simulink model "hdv_hydroelectropowertrain_model"  (R2026a)
settings: Solver=ode1be  StopTime=simulation_length  FixedStep=tsample  MaxStep=tsample
undefined symbols (not defined in the file): alpha, Apump, available_torque, Bpump, btheta_shaft, C1, consumption, Cpump, dp_lim, E0, E1, E2, E3, E_1, Elog, eta_v_m, eta_v_p, ki_dp_comp, ki_te_comp, kp_ctrl_m, kp_dp_comp, kp_te_comp, Kpump, load_blade_enable, Lpump, M, magnitude, Ncell, Npump, omega_e_rpm_ref, omega_l_max_rpm, q1Kalman, q2Kalman, q3Kalman, Qhr, R0, R1, R_tg, rKalman, rpm_base, rpm_consumption, simulation_length, tau_load, tau_load_max, Tc, torque_base, torque_consumption, torque_friction_base, tsample, v_track1_ref, v_track2_ref, valve_mmorifice_max, xv_m_max
libraries: fl_lib x383, nesl_utility x162, linear_swashplate_ctrl_lib x8, flexshaft_lib x5, bichamber_piston_lib x5, variable_displacement_motor_lib x4, variable_displacement_pump_lib x4, fixed_displacement_pump_lib x4, relief_valve_lib x4, inverse_shuttle_valve_lib x4, hydrostatic_threeway_valve_bichamber_piston_lib x4, hydrostatic_fourway_valve_bichamber_piston_lib x4
(part 3 of 8)

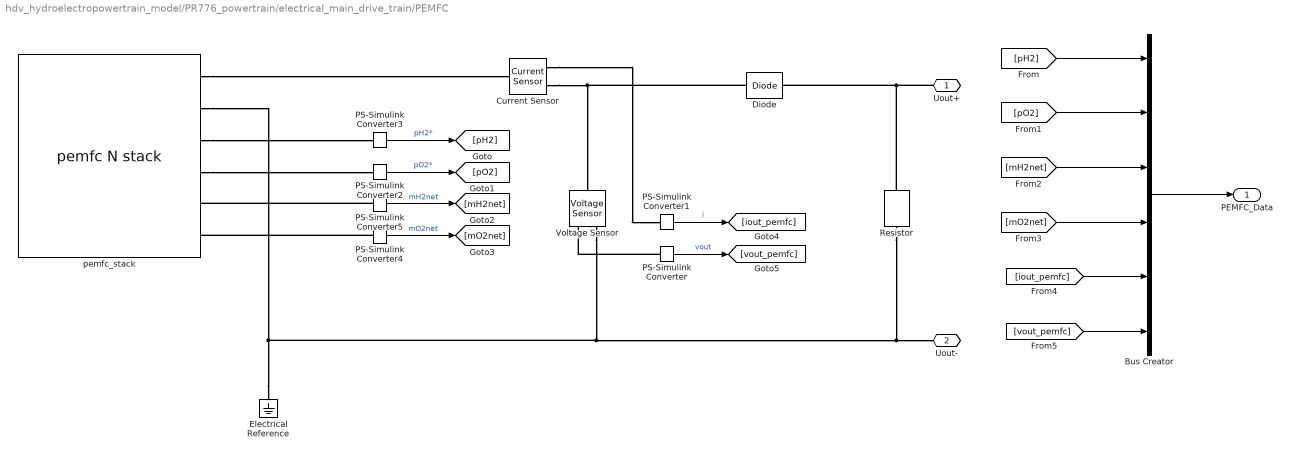
== system hdv_hydroelectropowertrain_model/PR776_powertrain/electrical_main_drive_train/PEMFC ==
  Bus Creator : BusCreator  Inputs=6
  Current Sensor : fl_lib/Electrical/Electrical Sensors/Current Sensor
  Diode : ee_lib/Semiconductors & Converters/Diode  ModelType=ee.enum.diode.modelType.pwl  TableType=ee.enum.diode.tableType.IfMat  IfMat=[.07, .12, .19, 1.75, 4.24, 7.32, 11.2; .16, .3, .72, 2.14, 5.02, 8.35, 13.12] A  VfMat=[.9, 1.15, 1.25, 1.5, 1.75, 2.17, 2.6, 2.85; .58, .68, .75, 1.1, 1.38, 1.77, 2.27, 2.7] V  TjVec=[25, 125] degC  VfVec=[.5, .7, .9, 1.3, 1.7, 2.1, 2.5] V  IfVec=[.1, .2, .5, 1, 2, 4, 7, 10] A  IrMat=[1e-06, 2e-06, 5e-06, 1e-05, 2.5e-05, 5e-05, .0001; 2e-06, 5e-06, 1e-05, 4e-05, 8e-05, .0002, .0005] A  VrMat=[10, 100, 200, 250, 300, 325, 350; 10, 70, 160, 220, 270, 300, 320] V  VrVec=[10, 20, 40, 50, 70, 80, 100] V  IrVec=[1e-06, 2e-06, 5e-06, 1e-05, 2e-05, 5e-05, .0001] A  Vf=0.6 V  Ron=0.3 Ohm  Goff=1e-8 S  prmExp=ee.enum.diode.expParam.useTwo  I12=[.0137, .545] A  V12=[.6, .7] V  RS=0 Ohm  Tmeas=25 degC  IS=1e-12 A  ec=1  I1=0.0137 A  V1=0.6 V  N_series=1  N_parallel=1  ZenerEnable=false  Rz=0.3 Ohm  BV=inf V  C_param=ee.enum.diode.capParam.fixed  CJ=5 pF  CJ0=5 pF  Vvec=[.1, 10, 100] V  Cvec=[3.5, 1, .4] pF  VJ=1 V  Mgrad=0.5  FC=0.5  Q_param=ee.enum.diode.recoveryParam.off  iRM=-7.15 A  iF=4 A  didt=-750 A/us  trr_factor=3  trr=115 ns  Qrr=1500 s*uA  Vr=-600 V  Ls=150 nH  Erec=0.03 J  TT=50 ns  tau=100 ns  T_param=ee.enum.diode.temperatureParam.off  Tdevice=25 degC  I1_T2=0.245 A  V1_T2=0.5 V  IS_T2=1.25e-7 A  Tmeas2=125 degC  XTI_param=ee.enum.diode.xtiParam.pn  XTI=3  EG_param=ee.enum.diode.egapParam.material_si  EG=1.11 eV  dBVdT=0 V/K  enable_fault_input=simscape.enum.onoff.off  i_specify=off  i_priority=None  i=0 A  i_nominal_specify=off  i_nominal_value=1  i_nominal_unit=A  v_specify=off  v_priority=None  v=0 V  v_nominal_specify=off  v_nominal_value=1  v_nominal_unit=V  v_capacitor_specify=off  v_capacitor_priority=None  v_capacitor=0 V  v_capacitor_nominal_specify=off  v_capacitor_nominal_value=1  v_capacitor_nominal_unit=V  Qj_specify=off  Qj_priority=High  Qj=0 C  Qj_nominal_specify=off  Qj_nominal_value=1  Qj_nominal_unit=C  i_diode_specify=off  i_diode_priority=None  i_diode=0 A  i_diode_nominal_specify=off  i_diode_nominal_value=1  i_diode_nominal_unit=A  v_diode_specify=off  v_diode_priority=None  v_diode=0 V  v_diode_nominal_specify=off  v_diode_nominal_value=1  v_diode_nominal_unit=V  i_capacitor_specify=off  i_capacitor_priority=None  i_capacitor=0 A  i_capacitor_nominal_specify=off  i_capacitor_nominal_value=1  i_capacitor_nominal_unit=A  fidelity_level=ee.enum.diode.fidelity.includeChargeDyn  rec_loss_model=ee.enum.diode.reverseRecoveryModel.fixed  ErecVal=0 J  scaleWithIandV=true  ErecMat=zeros(2, 3) J  ErecMat3D=zeros(2, 3, 2) J  TjrecVec=[298.15, 398.15] K  IfrecVec=[.1, 1, 10] A  IrecVal=10 A  VrecVal=10 V  VrecVec=[0, 100] V  tFilter=1 / 1000 / 100 s  thermal_network_parameterization=ee.enum.thermalNetworkTopology.junctionCase  Rth=[0, 10] K/W  Rth_Cauer=[1, 3, 10] K/W  Rth_Foster=[4, 6] K/W  thermal_mass_parameterization=ee.enum.thermalNetwork.timeconstant  thermal_mass=[0, 1] J/K  thermal_mass_Cauer=[.1, .3, 1] J/K  thermal_mass_Foster=[1.5, 3] J/K  thermal_time_constant=[0, 10] s  thermal_time_constant_Cauer=[1, 3, 10] s  thermal_time_constant_Foster=[6, 18] s  thermal_mass_initial_temperatures=[25, 25] degC  thermal_mass_initial_temperatures_Cauer=[25, 25, 25] degC  junction_thermal_mass=0.01 J/K  Tvec_initial_Foster=[25, 25, 25, 25] degC  no_thermal_network=0  junction_temperature_specify=off  junction_temperature_priority=None  junction_temperature=25 degC  junction_temperature_nominal_specify=off  junction_temperature_nominal_value=1  junction_temperature_nominal_unit=degC
  Electrical Reference : fl_lib/Electrical/Electrical Elements/Electrical Reference
  PS-Simulink Converter{,1..5} (6 alike) : nesl_utility/PS-Simulink Converter  PhysicalDomain=network_engine_domain  SubClassName=ps_output  LeftPortType=input  RightPortType=output  PseudoPeriodic=off  Frequencies=[]  VectorFormat=1-D array  Unit=inherit  AffineConversion=off
  Resistor : fl_lib/Electrical/Electrical Elements/Resistor  R=1e2 Ohm  i_specify=off  i_priority=None  i=0 A  i_nominal_specify=off  i_nominal_value=1  i_nominal_unit=A  v_specify=off  v_priority=None  v=0 V  v_nominal_specify=off  v_nominal_value=1  v_nominal_unit=V
  Voltage Sensor : fl_lib/Electrical/Electrical Sensors/Voltage Sensor
  pemfc_stack : pemfc_stack_lib/pemfc N stack  F=96487 s*A/mol  R=8.314 J/K/mol  T=298 K  DGibbs=285800 J/mol  n=2  Va=Va m^3  Vc=Vc m^3  tau_a=0.15 s  tau_c=0.15 s  p0=1e5 Pa  Ncells=Ncells  Rohm0=Rohm0 Ohm  Ract=Ract Ohm  Rconc=Rconc Ohm  Cdlc=Cdlc F  e_specify=off  e_priority=None  e=0 V  e_nominal_specify=off  e_nominal_unit=V  e_nominal_value=1  u_specify=off  u_priority=None  u=0 V  u_nominal_specify=off  u_nominal_unit=V  u_nominal_value=1  uc_specify=off  uc_priority=None  uc=0 V  uc_nominal_specify=off  uc_nominal_unit=V  uc_nominal_value=1  icell_specify=off  icell_priority=None  icell=0 A  icell_nominal_specify=off  icell_nominal_unit=A  icell_nominal_value=1  pH2_star_specify=off  pH2_star_priority=High  pH2_star=3  pH2_star_nominal_specify=off  pH2_star_nominal_unit=1  pH2_star_nominal_value=1  pO2_star_specify=off  pO2_star_priority=High  pO2_star=3  pO2_star_nominal_specify=off  pO2_star_nominal_unit=1  pO2_star_nominal_value=1  mH2_net_specify=off  mH2_net_priority=None  mH2_net=0 mol/s  mH2_net_nominal_specify=off  mH2_net_nominal_unit=mol/s  mH2_net_nominal_value=1  mO2_net_specify=off  mO2_net_priority=None  mO2_net=0 mol/s  mO2_net_nominal_specify=off  mO2_net_nominal_unit=mol/s  mO2_net_nominal_value=1  mask(pemfc N stack){}
  Uout+ : PMIOPort  Side=Right
  Uout- : PMIOPort  Port=2  Side=Right
  PEMFC_Data : Outport
  wires:
  PS-Simulink Converter2/1 -> [pO2]  "pO2*"
  PS-Simulink Converter1/1 -> [iout_pemfc]  "i"
  PS-Simulink Converter/1 -> [vout_pemfc]  "vout"
  PS-Simulink Converter3/1 -> [pH2]  "pH2*"
  PS-Simulink Converter5/1 -> [mH2net]  "mH2net"
  PS-Simulink Converter4/1 -> [mO2net]  "mO2net"
  Bus Creator/1 -> PEMFC_Data/1
  [pH2] -> Bus Creator/1
  [vout_pemfc] -> Bus Creator/6
  [pO2] -> Bus Creator/2
  [mH2net] -> Bus Creator/3
  [mO2net] -> Bus Creator/4
  [iout_pemfc] -> Bus Creator/5
  connections:
  pemfc_stack/RConn3 -- PS-Simulink Converter3/LConn1
  PS-Simulink Converter/LConn1 -- Voltage Sensor/RConn1
  pemfc_stack/RConn1 -- Current Sensor/LConn1
  pemfc_stack/RConn4 -- PS-Simulink Converter2/LConn1
  Electrical Reference/LConn1 -- Voltage Sensor/RConn2 -- Resistor/RConn1 -- Uout-/RConn1 -- pemfc_stack/RConn2
  Current Sensor/RConn1 -- PS-Simulink Converter1/LConn1
  PS-Simulink Converter4/LConn1 -- pemfc_stack/RConn6
  PS-Simulink Converter5/LConn1 -- pemfc_stack/RConn5
  Current Sensor/RConn2 -- Diode/LConn1 -- Voltage Sensor/LConn1
  Resistor/LConn1 -- Uout+/RConn1 -- Diode/RConn1

== system hdv_hydroelectropowertrain_model/PR776_powertrain/electrical_main_drive_train/battery_management ==
  vout(k) : Inport
  i(k) : Inport  Port=2
  Constant : Constant  Value=tsample
  Constant1 : Constant  Value=Qhr
  Constant2 : Constant  Value=q1Kalman
  Constant3 : Constant  Value=q2Kalman
  Constant4 : Constant  Value=q3Kalman
  Constant5 : Constant  Value=rKalman
  Constant6 : Constant  Value=tsample
  Constant7 : Constant  Value=Qhr
  Selector : Selector  InputPortWidth=3  IndexOptions=Index vector (dialog)  Indices=1  OutputSizes=1
  Unit Delay4 : UnitDelay  SampleTime=tsample
  kalman_observer_gains : MATLAB Function  TreatAsAtomicUnit=on  SystemSampleTime=tsample
  lithium-ion battery model : MATLAB Function  TreatAsAtomicUnit=on  SystemSampleTime=tsample
  SOC(k) : Outport
  vout_hat : Outport  Port=2
  wires:
  lithium-ion battery model/1(SOC) -> SOC(k)/1  "SOC"
  Constant6/1 -> kalman_observer_gains/2(ts)
  vout(k)/1 -> lithium-ion battery model/7(vout)
  kalman_observer_gains/2(l2) -> lithium-ion battery model/5(l2)
  Selector/1 -> Unit Delay4/1
  kalman_observer_gains/3(l3) -> lithium-ion battery model/6(l3)
  kalman_observer_gains/1(l1) -> lithium-ion battery model/4(l1)
  Constant7/1 -> kalman_observer_gains/8(Qhr)
  Constant1/1 -> lithium-ion battery model/3(Qhr)
  Constant5/1 -> kalman_observer_gains/7(r)
  Constant4/1 -> kalman_observer_gains/6(q3)
  Constant2/1 -> kalman_observer_gains/4(q1)
  Constant/1 -> lithium-ion battery model/2(ts)
  i(k)/1 -> kalman_observer_gains/1(iz), lithium-ion battery model/1(iz)
  lithium-ion battery model/3(x) -> Selector/1  "x(k+1|k)"
  Unit Delay4/1 -> kalman_observer_gains/3(z)  "x(k|k-1)"
  Constant3/1 -> kalman_observer_gains/5(q2)
  lithium-ion battery model/2(u) -> vout_hat/1  "vout_hat"

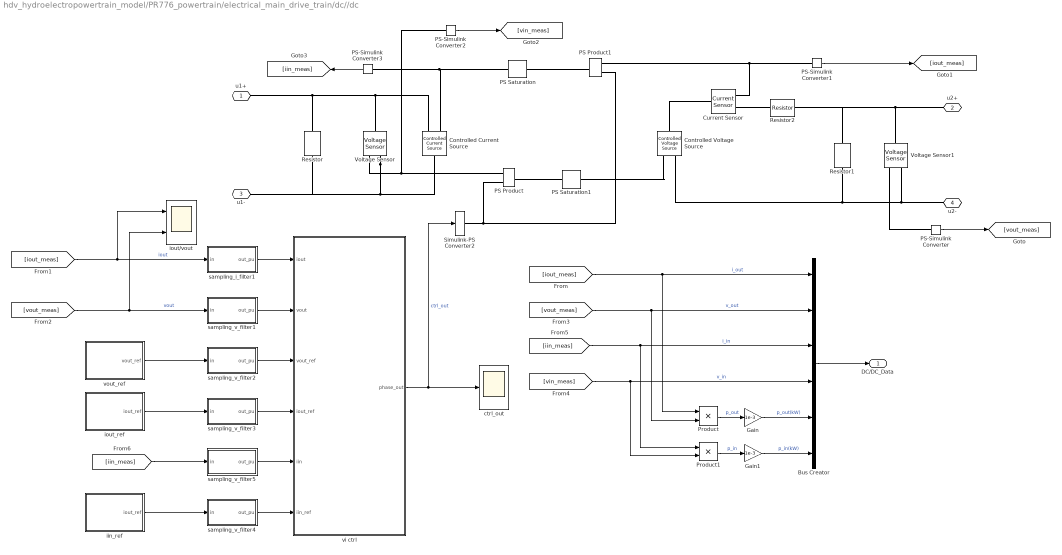
== system hdv_hydroelectropowertrain_model/PR776_powertrain/electrical_main_drive_train/dc//dc ==
  Bus Creator : BusCreator  Inputs=6
  Controlled Current Source : fl_lib/Electrical/Electrical Sources/Controlled Current Source
  Controlled Voltage Source : fl_lib/Electrical/Electrical Sources/Controlled Voltage Source
  Current Sensor : fl_lib/Electrical/Electrical Sensors/Current Sensor
  Gain : Gain  Gain=1e-3
  Gain1 : Gain  Gain=1e-3
  PS Product : fl_lib/Physical Signals/Functions/PS Product
  PS Product1 : fl_lib/Physical Signals/Functions/PS Product
  PS Saturation : fl_lib/Physical Signals/Nonlinear Operators/PS Saturation  upper_limit=inf A  lower_limit=-inf A  ZeroCross=true
  PS Saturation1 : fl_lib/Physical Signals/Nonlinear Operators/PS Saturation  upper_limit=inf V  lower_limit=-inf V  ZeroCross=true
  PS-Simulink Converter : nesl_utility/PS-Simulink Converter  PhysicalDomain=network_engine_domain  SubClassName=ps_output  LeftPortType=input  RightPortType=output  PseudoPeriodic=off  Frequencies=[]  VectorFormat=1-D array  Unit=inherit  AffineConversion=off
  PS-Simulink Converter1 : nesl_utility/PS-Simulink Converter  PhysicalDomain=network_engine_domain  SubClassName=ps_output  LeftPortType=input  RightPortType=output  PseudoPeriodic=off  Frequencies=[]  VectorFormat=1-D array  Unit=inherit  AffineConversion=on
  PS-Simulink Converter2 : nesl_utility/PS-Simulink Converter  PhysicalDomain=network_engine_domain  SubClassName=ps_output  LeftPortType=input  RightPortType=output  PseudoPeriodic=off  Frequencies=[]  VectorFormat=1-D array  Unit=inherit  AffineConversion=off
  PS-Simulink Converter3 : nesl_utility/PS-Simulink Converter  PhysicalDomain=network_engine_domain  SubClassName=ps_output  LeftPortType=input  RightPortType=output  PseudoPeriodic=off  Frequencies=[]  VectorFormat=1-D array  Unit=inherit  AffineConversion=off
  Product : Product
  Product1 : Product
  Resistor : fl_lib/Electrical/Electrical Elements/Resistor  R=1e4 Ohm  i_specify=off  i_priority=None  i=0 A  i_nominal_specify=off  i_nominal_value=1  i_nominal_unit=A  v_specify=off  v_priority=None  v=0 V  v_nominal_specify=off  v_nominal_value=1  v_nominal_unit=V
  Resistor1 : fl_lib/Electrical/Electrical Elements/Resistor  R=1e4 Ohm  i_specify=off  i_priority=None  i=0 A  i_nominal_specify=off  i_nominal_value=1  i_nominal_unit=A  v_specify=off  v_priority=None  v=0 V  v_nominal_specify=off  v_nominal_value=1  v_nominal_unit=V
  Resistor2 : fl_lib/Electrical/Electrical Elements/Resistor  R=5e-3 Ohm  i_specify=off  i_priority=None  i=0 A  i_nominal_specify=off  i_nominal_value=1  i_nominal_unit=A  v_specify=off  v_priority=None  v=0 V  v_nominal_specify=off  v_nominal_value=1  v_nominal_unit=V
  Simulink-PS Converter2 : nesl_utility/Simulink-PS Converter  PhysicalDomain=network_engine_domain  SubClassName=ps_input  LeftPortType=input  RightPortType=output  PseudoPeriodic=off  Frequencies=[]  NoiseDistribution=none  NoiseParameters=[]  Unit=1  AffineConversion=on  FilteringAndDerivatives=zero  SimscapeFilterOrder=2  InputFilterTimeConstant=tsample  UdotUserProvided=2
  Voltage Sensor : fl_lib/Electrical/Electrical Sensors/Voltage Sensor
  Voltage Sensor1 : fl_lib/Electrical/Electrical Sensors/Voltage Sensor
  ctrl_out : Scope
      settings: ActiveDisplayYMinimum=-0.85725  ActiveDisplayYMaximum=7.71521  DataLoggingVariableName=ScopeData5
  iin_ref : Subsystem
  iout/vout : Scope  NumInputPorts=2
      settings: ActiveDisplayYMinimum=-127511.09356  ActiveDisplayYMaximum=14266.88646
  iout_ref : Subsystem
  sampling_i_filter1 : Subsystem
  sampling_v_filter1 : Subsystem
  sampling_v_filter2 : Subsystem
  sampling_v_filter3 : Subsystem
  sampling_v_filter4 : Subsystem
  sampling_v_filter5 : Subsystem
  vi ctrl : Subsystem
  vout_ref : Subsystem
  u1+ : PMIOPort  Side=Left
  u2+ : PMIOPort  Port=2  Side=Right
  u1- : PMIOPort  Port=3  Side=Left
  u2- : PMIOPort  Port=4  Side=Right
  DC/DC_Data : Outport
  wires:
  vi ctrl/1(phase_out) -> Simulink-PS Converter2/1, ctrl_out/1  "ctrl_out"
  [iout_meas] -> iout/vout/1, sampling_i_filter1/1(in)  "iout"
  sampling_v_filter1/1(out_pu) -> vi ctrl/2(vout)
  sampling_v_filter2/1(out_pu) -> vi ctrl/3(vout_ref)
  [vout_meas] -> iout/vout/2, sampling_v_filter1/1(in)  "vout"
  sampling_i_filter1/1(out_pu) -> vi ctrl/1(iout)
  vout_ref/1(vout_ref) -> sampling_v_filter2/1(in)
  PS-Simulink Converter/1 -> [vout_meas]
  iout_ref/1(iout_ref) -> sampling_v_filter3/1(in)
  sampling_v_filter3/1(out_pu) -> vi ctrl/4(iout_ref)
  Bus Creator/1 -> DC/DC_Data/1
  [iout_meas] -> Product/1, Bus Creator/1  "i_out"
  [vout_meas] -> Product/2, Bus Creator/2  "v_out"
  PS-Simulink Converter2/1 -> [vin_meas]
  [vin_meas] -> Product1/2, Bus Creator/4  "v_in"
  PS-Simulink Converter3/1 -> [iin_meas]
  [iin_meas] -> Product1/1, Bus Creator/3  "i_in"
  Product/1 -> Gain/1  "p_out"
  Product1/1 -> Gain1/1  "p_in"
  Gain/1 -> Bus Creator/5  "p_out(kW)"
  Gain1/1 -> Bus Creator/6  "p_in(kW)"
  PS-Simulink Converter1/1 -> [iout_meas]
  iin_ref/1(iout_ref) -> sampling_v_filter4/1(in)
  sampling_v_filter4/1(out_pu) -> vi ctrl/6(iin_ref)
  sampling_v_filter5/1(out_pu) -> vi ctrl/5(iin)
  [iin_meas] -> sampling_v_filter5/1(in)
  connections:
  Simulink-PS Converter2/RConn1 -- PS Product/LConn2 -- PS Product1/LConn1
  Current Sensor/RConn1 -- PS-Simulink Converter1/LConn1 -- PS Product1/LConn2
  Voltage Sensor/RConn1 -- PS-Simulink Converter2/LConn1 -- PS Product/LConn1
  Voltage Sensor/RConn2 -- Resistor/RConn1 -- u1-/RConn1 -- Controlled Current Source/LConn1
  Controlled Voltage Source/RConn2 -- Resistor1/RConn1 -- Voltage Sensor1/RConn2 -- u2-/RConn1
  Controlled Voltage Source/LConn1 -- Current Sensor/LConn1
  PS Product1/RConn1 -- PS Saturation/LConn1
  PS Product/RConn1 -- PS Saturation1/LConn1
  Voltage Sensor1/RConn1 -- PS-Simulink Converter/LConn1
  PS Saturation/RConn1 -- PS-Simulink Converter3/LConn1 -- Controlled Current Source/RConn1
  PS Saturation1/RConn1 -- Controlled Voltage Source/RConn1
  Voltage Sensor1/LConn1 -- Resistor2/RConn1 -- Resistor1/LConn1 -- u2+/RConn1
  Resistor/LConn1 -- Voltage Sensor/LConn1 -- Controlled Current Source/RConn2 -- u1+/RConn1
  Resistor2/LConn1 -- Current Sensor/RConn2

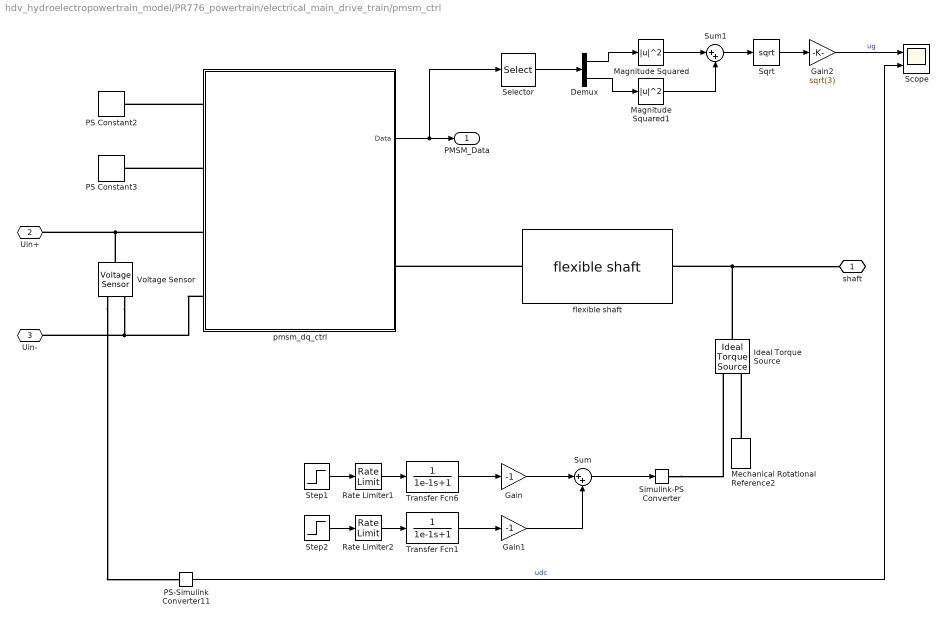
== system hdv_hydroelectropowertrain_model/PR776_powertrain/electrical_main_drive_train/pmsm_ctrl ==
  Demux : Demux  Outputs=2
  Gain : Gain  Gain=-1
  Gain1 : Gain  Gain=-1
  Gain2 : Gain  Gain=sqrt(3)
  Ideal Torque Source : fl_lib/Mechanical/Mechanical Sources/Ideal Torque Source
  Magnitude Squared : Math  Operator=magnitude^2
  Magnitude Squared1 : Math  Operator=magnitude^2
  Mechanical Rotational Reference2 : fl_lib/Mechanical/Rotational Elements/Mechanical Rotational Reference
  PS Constant2 : fl_lib/Physical Signals/Sources/PS Constant  constant=1800 rpm
  PS Constant3 : fl_lib/Physical Signals/Sources/PS Constant  constant=1140 N*m
  PS-Simulink Converter11 : nesl_utility/PS-Simulink Converter  PhysicalDomain=network_engine_domain  SubClassName=ps_output  LeftPortType=input  RightPortType=output  PseudoPeriodic=off  Frequencies=[]  VectorFormat=1-D array  Unit=V  AffineConversion=on
  Rate Limiter1 : RateLimiter  RisingSlewLimit=500  FallingSlewLimit=-500  SampleTimeMode=inherited
  Rate Limiter2 : RateLimiter  RisingSlewLimit=500  FallingSlewLimit=-500  SampleTimeMode=inherited
  Scope : Scope  NumInputPorts=2
      settings: SampleTime=tsample  ActiveDisplayYMinimum=-91.13418  ActiveDisplayYMaximum=820.20758
  Selector : Selector  InputPortWidth=13  IndexOptions=Index vector (dialog)  Indices=[11 12]  OutputSizes=1
  Simulink-PS Converter : nesl_utility/Simulink-PS Converter  PhysicalDomain=network_engine_domain  SubClassName=ps_input  LeftPortType=input  RightPortType=output  PseudoPeriodic=off  Frequencies=[]  NoiseDistribution=none  NoiseParameters=[]  Unit=N*m  AffineConversion=on  FilteringAndDerivatives=provide  SimscapeFilterOrder=1  InputFilterTimeConstant=0.001  UdotUserProvided=0
  Sqrt : Sqrt
  Step1 : Step  Time=simulation_length/5  FinalValue=1140/20  SampleTime=0
  Step2 : Step  Time=simulation_length*2/5  FinalValue=1140/20  SampleTime=0
  Sum : Sum  Inputs=|++
  Sum1 : Sum  Inputs=|++
  Transfer Fcn1 : TransferFcn  Denominator=[1e-1 1]
  Transfer Fcn6 : TransferFcn  Denominator=[1e-1 1]
  Voltage Sensor : fl_lib/Electrical/Electrical Sensors/Voltage Sensor
  flexible shaft : flexshaft_lib/flexible shaft  b1=1e-2 N*m/(rad/s)  J1=1.25/5 kg*m^2  b2=1e-2 N*m/(rad/s)  J2=1.25/5 kg*m^2  b_theta=1 N*m/(rad/s)  k_theta=1e5 N*m/rad  w_1_specify=off  w_1_priority=None  w_1=0 rad/s  w_1_nominal_specify=off  w_1_nominal_value=1  w_1_nominal_unit=rad/s  w_2_specify=off  w_2_priority=None  w_2=0 rad/s  w_2_nominal_specify=off  w_2_nominal_value=1  w_2_nominal_unit=rad/s  t_1_specify=off  t_1_priority=None  t_1=0 N*m  t_1_nominal_specify=off  t_1_nominal_value=1  t_1_nominal_unit=N*m  t_2_specify=off  t_2_priority=None  t_2=0 N*m  t_2_nominal_specify=off  t_2_nominal_value=1  t_2_nominal_unit=N*m  t_theta_specify=off  t_theta_priority=None  t_theta=0 N*m  t_theta_nominal_specify=off  t_theta_nominal_value=1  t_theta_nominal_unit=N*m
  pmsm_dq_ctrl : Subsystem  mask{control_mode=Speed Mode, torque_limitation=Torque limited from torque ref, polepairs=8, poles_unit=1, omega_m_max=2700, omega_m_max_unit=rpm, omega_m_nom=1800, omega_m_nom_unit=rpm, tau_nom=1140, tau_nom_unit=N*m, Rs=0.016, Rs_unit=Ohm, Ld=0.000274, Ld_unit=H, Lq=0.000263, Lq_unit=H, Ke=0.206, Ke_unit=V*s, Kt=3.35, Kt_unit=N*m/Arms, J=0.2, J_unit=kg*m^2, b=0.02, b_unit=N*m/(rad/s), kp_w=4, ki_w=35, kp_i=0.5, ki_i=18, kp_fw=0.1, ki_fw=2}
      mask prompts: control_mode "Enable Speed Mode"; torque_limitation "Enable Torque Limitation"; polepairs "Number of motor pole pairs"; omega_m_max "Maximum Speed"; omega_m_nom "Nominal Speed"; tau_nom "Nominal Torque"; Ke "Voltage Constant"; Kt "Torque Constant"; J "Rotor Inertia"; b "Viscosity"; kp_w "Proportional Speed Ctrl Gain"; ki_w "Integral Speed Ctrl Gain"; kp_i "Proportional Current Ctrl Gain"; ki_i "Integral Current Ctrl Gain"; kp_fw "Proportional Field Weakening Ctrl Gain"; ki_fw "Integral Field Weakening Ctrl Gain"
      mask init:
      | cm = get_param(gcb,'control_mode');
      | tl = get_param(gcb,'torque_limitation');
      | 
      | poles = 2*polepairs;
      | if Ke > 0
      |     phi_m = Ke;
      | elseif Kt > 0
      |     phi_m = Kt*sqrt(2)/3/polepairs;
      | else
      |     phi_m = 1;
      | end
      | 
      | omega_bez = omega_m_nom*polepairs/60*2*pi;
      | ubez = phi_m*omega_bez;
      | 
      | if Kt > 0
      |     ibez = tau_nom/Kt*sqrt(2);
      | else
      |     ibez = 2*tau_nom/3/p/psi_m;
      | end
      | phi_m_unit = 'V*s';
      | ubez_unit = 'V';
      | ibez_unit = 'A';
      | omega_bez_unit = 'rad/s';
      | 
      | motor = [gcb, '/pmsm_dq2'];
      | 
      | set_param([motor],'emf_nom','ubez');
      | set_param([motor],'emf_nom_unit',ubez_unit);
      | set_param([motor],'i_nom','ibez');
      | set_param([motor],'i_nom_unit',ibez_unit);
      | set_param([motor],'omega_nom','omega_bez');
      | set_param([motor],'omega_nom_unit',omega_bez_unit);
      | set_param([motor],'poles','poles');
      | set_param([motor],'poles_unit',poles_unit);
      | set_param([motor],'Rs','Rs');
      | set_param([motor],'Rs_unit',Rs_unit);
      | set_param([motor],'Ld','Ld');
      | set_param([motor],'Ld_unit',Ld_unit);
      | set_param([motor],'Lq','Lq');
      | set_param([motor],'Lq_unit',Lq_unit);
      | set_param([motor],'phi_m','phi_m');
      | set_param([motor],'phi_m_unit',phi_m_unit);
      | set_param([motor],'J','J');
      | set_param([motor],'J_unit',J_unit);
      | set_param([motor],'b','b');
      | set_param([motor],'b_unit',b_unit);
      | 
      | controller = [gcb, '/pmsm dq controller'];
      | set_param([controller],'emf_nom','ubez');
      | set_param([controller],'emf_nom_unit',ubez_unit);
      | set_param([controller],'i_nom','ibez');
      | set_param([controller],'i_nom_unit',ibez_unit);
      | set_param([controller],'omega_m_nom','omega_bez');
      | set_param([controller],'omega_m_nom_unit',omega_bez_unit);
      | set_param([controller],'poles','poles');
      | set_param([controller],'Rs','Rs');
      | set_param([controller],'Rs_unit',Rs_unit);
      | set_param([controller],'Ld','Ld');
      | set_param([controller],'Ld_unit',Ld_unit);
      | set_param([controller],'Lq','Lq');
      | set_param([controller],'Lq_unit',Lq_unit);
      | set_param([controller],'phi_m','phi_m');
      | set_param([controller],'phi_m_unit',phi_m_unit);
      | set_param([controller],'kp_w','kp_w');
      | set_param([controller],'ki_w','ki_w');
      | set_param([controller],'kp_i','kp_i');
      | set_param([controller],'ki_i','ki_i');
      | set_param([controller],'kp_fw','kp_fw');
      | set_param([controller],'ki_fw','ki_fw');
      | switch cm
      |     case 'Speed Mode'
      |         set_param([controller],'Speed_mode','simscape.enum.onoff.on');
      |     case 'Torque Mode'
      |         set_param([controller],'Speed_mode','simscape.enum.onoff.off');
      | end
      | switch tl
      |     case 'Torque limited from torque ref'
      |         set_param([controller],'TorqueLim','simscape.enum.onoff.on');
      |     case 'Torque unlimited'
      |         set_param([controller],'TorqueLim','simscape.enum.onoff.off');
      | end
      mask Help: eval('open \documentation\pmsm_ctrl_i.pdf')
      mask TypeOptions control_mode: Speed Mode | Torque Mode
      mask TypeOptions torque_limitation: Torque limited from torque ref | Torque unlimited
      mask TypeOptions poles_unit: 1
      mask TypeOptions omega_m_max_unit: rpm
      mask TypeOptions omega_m_nom_unit: rpm
      mask TypeOptions tau_nom_unit: N*m
      mask TypeOptions Rs_unit: Ohm
      mask TypeOptions Ld_unit: H
      mask TypeOptions Lq_unit: H
      mask TypeOptions Ke_unit: V*s
      mask TypeOptions Kt_unit: N*m/Arms
      mask TypeOptions J_unit: kg*m^2
      mask TypeOptions b_unit: N*m/(rad/s)
      mask DialogControl ModeofOperation Prompt: Mode of Operation
      mask DialogControl MotorParameters Prompt: Motor Parameters
      mask DialogControl ControlParameters Prompt: Control Parameters
      mask Display:
      | % Icon = 'C:\Users\dbagn\Dropbox\davide\11_matlab\11.73 HydraulicComponents\IM.jpg'
      | 
      | 
      | modelname = [gcb];
      | % image(imread("library\+pmsm_dq2\pmsm_drawing_mask.png"));
      | 
      | color('red')
      | port_label('lconn',1,'Speed Reference');
      | color('red')
      | port_label('lconn',2,'Maximum Torque');
      | color('blue')
      | port_label('lconn',3,'Uin+');
      | color('blue')
      | port_label('lconn',4,'Uin-');
      | color('black')
      | port_label('output',1,'PMSM data');
      | color('green')
      | port_label('rconn',1,'D')
  shaft : PMIOPort  Side=Right
  Uin+ : PMIOPort  Port=2  Side=Left
  Uin- : PMIOPort  Port=3  Side=Left
  PMSM_Data : Outport
  wires:
  Transfer Fcn6/1 -> Gain/1
  Step1/1 -> Rate Limiter1/1
  Rate Limiter1/1 -> Transfer Fcn6/1
  pmsm_dq_ctrl/1(Data) -> Selector/1, PMSM_Data/1
  Gain/1 -> Sum/1
  Rate Limiter2/1 -> Transfer Fcn1/1
  Step2/1 -> Rate Limiter2/1
  Sum/1 -> Simulink-PS Converter/1
  Transfer Fcn1/1 -> Gain1/1
  Gain1/1 -> Sum/2
  Selector/1 -> Demux/1
  Demux/1 -> Magnitude Squared/1
  Demux/2 -> Magnitude Squared1/1
  Magnitude Squared/1 -> Sum1/1
  Magnitude Squared1/1 -> Sum1/2
  Sum1/1 -> Sqrt/1
  Sqrt/1 -> Gain2/1
  PS-Simulink Converter11/1 -> Scope/2  "udc"
  Gain2/1 -> Scope/1  "ug"
  connections:
  Mechanical Rotational Reference2/LConn1 -- Ideal Torque Source/RConn2
  Ideal Torque Source/LConn1 -- shaft/RConn1 -- flexible shaft/RConn1
  Simulink-PS Converter/RConn1 -- Ideal Torque Source/RConn1
  flexible shaft/LConn1 -- pmsm_dq_ctrl/RConn1
  Voltage Sensor/LConn1 -- pmsm_dq_ctrl/LConn3 -- Uin+/RConn1
  Voltage Sensor/RConn2 -- pmsm_dq_ctrl/LConn4 -- Uin-/RConn1
  Voltage Sensor/RConn1 -- PS-Simulink Converter11/LConn1
  pmsm_dq_ctrl/LConn1 -- PS Constant2/RConn1
  pmsm_dq_ctrl/LConn2 -- PS Constant3/RConn1

== system hdv_hydroelectropowertrain_model/PR776_powertrain/front_blade_model/blade_height ==
  Rate Limiter : RateLimiter  RisingSlewLimit=0.02  FallingSlewLimit=-0.02  SampleTimeMode=inherited
  Saturation : Saturate  UpperLimit=1  LowerLimit=0
  Step5 : Step  Time=simulation_length/3  FinalValue=0.5  SampleTime=0
  Transfer Fcn : TransferFcn  Denominator=[1e-2 1]
  blade_height : Outport
  wires:
  Saturation/1 -> Transfer Fcn/1
  Transfer Fcn/1 -> blade_height/1
  Rate Limiter/1 -> Saturation/1
  Step5/1 -> Rate Limiter/1

== system hdv_hydroelectropowertrain_model/PR776_powertrain/front_blade_model/hose ==
  Constant Area Hydraulic Orifice : fl_lib/Hydraulic/Hydraulic Elements/Constant Area Hydraulic Orifice  area=1e-8 m^2  C_d=0.7  lam_spec=1  B_lam=0.999  Re_cr=12  q_specify=off  q_priority=None  q=0.001 m^3/s  q_nominal_specify=off  q_nominal_value=1  q_nominal_unit=m^3/s  p_specify=off  p_priority=None  p=0 Pa  p_nominal_specify=off  p_nominal_value=1  p_nominal_unit=Pa
  Constant Area Hydraulic Orifice1 : fl_lib/Hydraulic/Hydraulic Elements/Constant Area Hydraulic Orifice  area=1e-8 m^2  C_d=0.7  lam_spec=1  B_lam=0.999  Re_cr=12  q_specify=off  q_priority=None  q=0.001 m^3/s  q_nominal_specify=off  q_nominal_value=1  q_nominal_unit=m^3/s  p_specify=off  p_priority=None  p=0 Pa  p_nominal_specify=off  p_nominal_value=1  p_nominal_unit=Pa
  Hydraulic Flow Rate Sensor3 : fl_lib/Hydraulic/Hydraulic Sensors/Hydraulic Flow Rate Sensor
  Hydraulic Flow Rate Source : fl_lib/Hydraulic/Hydraulic Sources/Hydraulic Flow Rate Source
  Hydraulic Pressure Sensor2 : fl_lib/Hydraulic/Hydraulic Sensors/Hydraulic Pressure Sensor
  Hydraulic Pressure Source : fl_lib/Hydraulic/Hydraulic Sources/Hydraulic Pressure Source
  Hydraulic Reference : fl_lib/Hydraulic/Hydraulic Elements/Hydraulic Reference
  PS Gain : fl_lib/Physical Signals/Functions/PS Gain  gain=1 Pa
  PS Gain1 : fl_lib/Physical Signals/Functions/PS Gain  gain=1 Pa^-1
  PS Gain2 : fl_lib/Physical Signals/Functions/PS Gain  gain=1 m^3/s
  PS Gain3 : fl_lib/Physical Signals/Functions/PS Gain  gain=1 m^-3*s
  PS Transfer Function : fl_lib/Physical Signals/Linear Operators/PS Transfer Function  transfer_function_type=foundation.enum.transfer_function_type.lag  T=0.1 s  T1=2 s  T2=1 s  reset_method=foundation.enum.IntegratorResetSpec.None  initial_condition_spec=foundation.enum.IntegratorICSpec.Internal  y0=0
  PS Transfer Function1 : fl_lib/Physical Signals/Linear Operators/PS Transfer Function  transfer_function_type=foundation.enum.transfer_function_type.lag  T=0.1 s  T1=2 s  T2=1 s  reset_method=foundation.enum.IntegratorResetSpec.None  initial_condition_spec=foundation.enum.IntegratorICSpec.Internal  y0=0
  A : PMIOPort  Side=Left
  ps : PMIOPort  Port=2  Side=Right
  B : PMIOPort  Port=3  Side=Left
  pt : PMIOPort  Port=4  Side=Right
  connections:
  ps/RConn1 -- Constant Area Hydraulic Orifice1/LConn1 -- Hydraulic Flow Rate Sensor3/RConn2
  PS Gain2/RConn1 -- Hydraulic Flow Rate Source/RConn1
  Hydraulic Flow Rate Sensor3/RConn1 -- PS Gain3/LConn1
  Hydraulic Flow Rate Sensor3/LConn1 -- Hydraulic Pressure Source/LConn1
  Hydraulic Pressure Source/RConn1 -- PS Gain/RConn1
  PS Gain1/LConn1 -- Hydraulic Pressure Sensor2/RConn2
  Hydraulic Pressure Source/RConn2 -- Hydraulic Pressure Sensor2/RConn1 -- Constant Area Hydraulic Orifice/RConn1 -- B/RConn1 -- Hydraulic Flow Rate Source/LConn1 -- Constant Area Hydraulic Orifice1/RConn1 -- Hydraulic Reference/LConn1 -- pt/RConn1
  PS Transfer Function1/RConn1 -- PS Gain2/LConn1
  PS Transfer Function/RConn1 -- PS Gain/LConn1
  A/RConn1 -- Constant Area Hydraulic Orifice/LConn1 -- Hydraulic Pressure Sensor2/LConn1 -- Hydraulic Flow Rate Source/RConn2
  PS Gain3/RConn1 -- PS Transfer Function1/LConn1
  PS Gain1/RConn1 -- PS Transfer Function/LConn1

== system hdv_hydroelectropowertrain_model/PR776_powertrain/front_blade_model/piston_tilt ==
  ref : Inport
  PS-Simulink Converter{1..5,7,9} (7 alike) : nesl_utility/PS-Simulink Converter  PhysicalDomain=network_engine_domain  SubClassName=ps_output  LeftPortType=input  RightPortType=output  PseudoPeriodic=off  Frequencies=[]  VectorFormat=1-D array  Unit=inherit  AffineConversion=off
  bichamber piston A : bichamber_piston_lib/bichamber piston  A1=8e-3 m^2  A2=8e-3 m^2  Lp=1 m  mp=35 kg  kp=0 N/m  bp=1e3 N/(m/s)  V0=12 l  q1_specify=off  q1_priority=None  q1=0 m^3/s  q1_nominal_specify=off  q1_nominal_value=1  q1_nominal_unit=m^3/s  q2_specify=off  q2_priority=None  q2=0 m^3/s  q2_nominal_specify=off  q2_nominal_value=1  q2_nominal_unit=m^3/s  p1_specify=off  p1_priority=High  p1=0 bar  p1_nominal_specify=off  p1_nominal_value=1  p1_nominal_unit=bar  p2_specify=off  p2_priority=High  p2=0 bar  p2_nominal_specify=off  p2_nominal_value=1  p2_nominal_unit=bar  fp_specify=off  fp_priority=None  fp=0 N  fp_nominal_specify=off  fp_nominal_value=1  fp_nominal_unit=N  vp_specify=off  vp_priority=None  vp=0 m/s  vp_nominal_specify=off  vp_nominal_value=1  vp_nominal_unit=m/s  xp_specify=off  xp_priority=High  xp=0 m  xp_nominal_specify=off  xp_nominal_value=1  xp_nominal_unit=m
  blade_tilt_model : Subsystem
  controller : Subsystem
  flow : Scope  NumInputPorts=2
      settings: ActiveDisplayYMinimum=-390.093  ActiveDisplayYMaximum=390.1347
  fm : Scope
      settings: ActiveDisplayYMinimum=-1966.05122  ActiveDisplayYMaximum=2078.06244  DataLoggingVariableName=ScopeData2
  fourway_threeland_valve : fourway_threeland_valve_lib/fourway_threeland_valve  xv_max=valve_mmorifice_max mm  q1_specify=off  q1_priority=None  q1=0 m^3/s  q1_nominal_specify=off  q1_nominal_unit=m^3/s  q1_nominal_value=1  q2_specify=off  q2_priority=None  q2=0 m^3/s  q2_nominal_specify=off  q2_nominal_unit=m^3/s  q2_nominal_value=1  qin_specify=off  qin_priority=None  qin=0 m^3/s  qin_nominal_specify=off  qin_nominal_unit=m^3/s  qin_nominal_value=1  qout_specify=off  qout_priority=None  qout=0 m^3/s  qout_nominal_specify=off  qout_nominal_unit=m^3/s  qout_nominal_value=1  p1_specify=off  p1_priority=None  p1=0 bar  p1_nominal_specify=off  p1_nominal_unit=bar  p1_nominal_value=1  p2_specify=off  p2_priority=None  p2=0 bar  p2_nominal_specify=off  p2_nominal_unit=bar  p2_nominal_value=1  ps_specify=off  ps_priority=None  ps=0 bar  ps_nominal_specify=off  ps_nominal_unit=bar  ps_nominal_value=1  pt_specify=off  pt_priority=None  pt=0 bar  pt_nominal_specify=off  pt_nominal_unit=bar  pt_nominal_value=1
  p1/p2 : Scope  NumInputPorts=2
      settings: ActiveDisplayYMinimum=121.45609  ActiveDisplayYMaximum=128.13349  DataLoggingVariableName=ScopeData4
  xp/vp : Scope  NumInputPorts=2
      settings: ActiveDisplayYMinimum=-0.06251  ActiveDisplayYMaximum=0.56255
  xp_re/xp : Scope  NumInputPorts=2
      settings: ActiveDisplayYMinimum=-0.12375  ActiveDisplayYMaximum=1.11375  DataLoggingVariableName=ScopeData7
  ps : PMIOPort  Side=Left
  pt : PMIOPort  Port=2  Side=Left
  load : PMIOPort  Port=3  Side=Right
  wires:
  ref/1 -> blade_tilt_model/1(xp_ref), xp_re/xp/1, controller/1(ref)
  PS-Simulink Converter3/1 -> p1/p2/1  "p1"
  PS-Simulink Converter7/1 -> controller/2(xp), xp_re/xp/2, xp/vp/1  "xp"
  PS-Simulink Converter4/1 -> flow/2  "q2"
  PS-Simulink Converter9/1 -> xp/vp/2  "vp"
  PS-Simulink Converter5/1 -> p1/p2/2  "p2"
  PS-Simulink Converter1/1 -> flow/1  "q1"
  PS-Simulink Converter2/1 -> fm/1  "fm"
  connections:
  bichamber piston A/RConn3 -- PS-Simulink Converter9/LConn1
  bichamber piston A/LConn2 -- fourway_threeland_valve/RConn2
  bichamber piston A/LConn1 -- fourway_threeland_valve/RConn1
  bichamber piston A/RConn2 -- PS-Simulink Converter7/LConn1
  bichamber piston A/RConn4 -- PS-Simulink Converter2/LConn1
  bichamber piston A/RConn5 -- PS-Simulink Converter1/LConn1
  bichamber piston A/RConn6 -- PS-Simulink Converter4/LConn1
  bichamber piston A/RConn7 -- PS-Simulink Converter3/LConn1
  bichamber piston A/RConn8 -- PS-Simulink Converter5/LConn1
  ps/RConn1 -- fourway_threeland_valve/LConn2
  pt/RConn1 -- fourway_threeland_valve/LConn3
  fourway_threeland_valve/LConn1 -- controller/RConn1
  blade_tilt_model/LConn1 -- bichamber piston A/RConn1
  load/RConn1 -- blade_tilt_model/RConn1

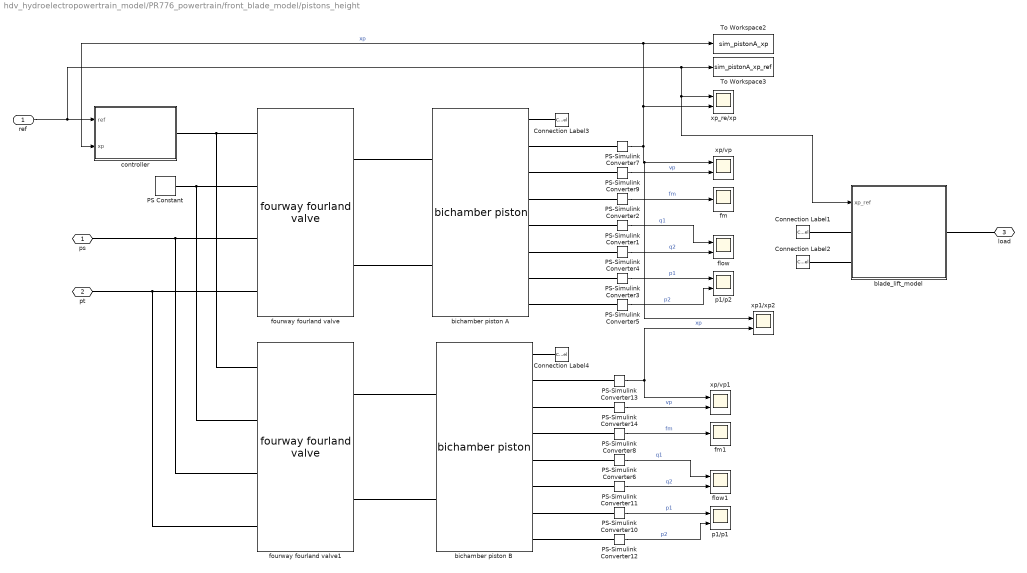
== system hdv_hydroelectropowertrain_model/PR776_powertrain/front_blade_model/pistons_height ==
  ref : Inport
  Connection Label1 : ConnectionLabel  Label=A
  Connection Label2 : ConnectionLabel  Label=B
  Connection Label3 : ConnectionLabel  Label=A
  Connection Label4 : ConnectionLabel  Label=B
  PS Constant : fl_lib/Physical Signals/Sources/PS Constant  constant=0 mm
  PS-Simulink Converter{1..14} (14 alike) : nesl_utility/PS-Simulink Converter  PhysicalDomain=network_engine_domain  SubClassName=ps_output  LeftPortType=input  RightPortType=output  PseudoPeriodic=off  Frequencies=[]  VectorFormat=1-D array  Unit=inherit  AffineConversion=off
  To Workspace2 : ToWorkspace  VariableName=sim_pistonA_xp  SampleTime=Tc
      settings: MaxDataPoints=Nc
  To Workspace3 : ToWorkspace  VariableName=sim_pistonA_xp_ref  SampleTime=Tc
      settings: MaxDataPoints=Nc
  bichamber piston A : bichamber_piston_lib/bichamber piston  A1=8e-3 m^2  A2=8e-3 m^2  Lp=1 m  mp=35 kg  kp=0 N/m  bp=1e3 N/(m/s)  V0=12 l  q1_specify=off  q1_priority=None  q1=0 m^3/s  q1_nominal_specify=off  q1_nominal_value=1  q1_nominal_unit=m^3/s  q2_specify=off  q2_priority=None  q2=0 m^3/s  q2_nominal_specify=off  q2_nominal_value=1  q2_nominal_unit=m^3/s  p1_specify=off  p1_priority=High  p1=0 bar  p1_nominal_specify=off  p1_nominal_value=1  p1_nominal_unit=bar  p2_specify=off  p2_priority=High  p2=125 bar  p2_nominal_specify=off  p2_nominal_value=1  p2_nominal_unit=bar  fp_specify=off  fp_priority=None  fp=0 N  fp_nominal_specify=off  fp_nominal_value=1  fp_nominal_unit=N  vp_specify=off  vp_priority=None  vp=0 m/s  vp_nominal_specify=off  vp_nominal_value=1  vp_nominal_unit=m/s  xp_specify=off  xp_priority=High  xp=0 m  xp_nominal_specify=off  xp_nominal_value=1  xp_nominal_unit=m
  bichamber piston B : bichamber_piston_lib/bichamber piston  A1=8e-3 m^2  A2=8e-3 m^2  Lp=1 m  mp=35 kg  kp=0 N/m  bp=1e3 N/(m/s)  V0=12 l  q1_specify=off  q1_priority=None  q1=0 m^3/s  q1_nominal_specify=off  q1_nominal_value=1  q1_nominal_unit=m^3/s  q2_specify=off  q2_priority=None  q2=0 m^3/s  q2_nominal_specify=off  q2_nominal_value=1  q2_nominal_unit=m^3/s  p1_specify=off  p1_priority=High  p1=0 bar  p1_nominal_specify=off  p1_nominal_value=1  p1_nominal_unit=bar  p2_specify=off  p2_priority=High  p2=125 bar  p2_nominal_specify=off  p2_nominal_value=1  p2_nominal_unit=bar  fp_specify=off  fp_priority=None  fp=0 N  fp_nominal_specify=off  fp_nominal_value=1  fp_nominal_unit=N  vp_specify=off  vp_priority=None  vp=0 m/s  vp_nominal_specify=off  vp_nominal_value=1  vp_nominal_unit=m/s  xp_specify=off  xp_priority=High  xp=0 m  xp_nominal_specify=off  xp_nominal_value=1  xp_nominal_unit=m
  blade_lift_model : Subsystem
  controller : Subsystem
  flow : Scope  NumInputPorts=2
      settings: ActiveDisplayYMinimum=-1  ActiveDisplayYMaximum=1
  flow1 : Scope  NumInputPorts=2
      settings: ActiveDisplayYMinimum=-7061.36378  ActiveDisplayYMaximum=62073.30078
  fm : Scope
      settings: SampleTime=tsample  ActiveDisplayYMinimum=-3786.84749  ActiveDisplayYMaximum=34081.62739  DataLoggingVariableName=ScopeData2
  fm1 : Scope
      settings: ActiveDisplayYMinimum=-88.79535  ActiveDisplayYMaximum=247.97012  DataLoggingVariableName=ScopeData2
  fourway fourland valve : fourway_fourland_valve_lib/fourway fourland valve  xv_max=valve_mmorifice_max mm  ps_specify=off  ps_priority=None  ps=0 bar  ps_nominal_specify=off  ps_nominal_unit=bar  ps_nominal_value=1  pt_specify=off  pt_priority=None  pt=0 bar  pt_nominal_specify=off  pt_nominal_unit=bar  pt_nominal_value=1  q1_specify=off  q1_priority=None  q1=0 m^3/s  q1_nominal_specify=off  q1_nominal_unit=m^3/s  q1_nominal_value=1  q2_specify=off  q2_priority=None  q2=0 m^3/s  q2_nominal_specify=off  q2_nominal_unit=m^3/s  q2_nominal_value=1  q3_specify=off  q3_priority=None  q3=0 m^3/s  q3_nominal_specify=off  q3_nominal_unit=m^3/s  q3_nominal_value=1  q4_specify=off  q4_priority=None  q4=0 m^3/s  q4_nominal_specify=off  q4_nominal_unit=m^3/s  q4_nominal_value=1  q5_specify=off  q5_priority=None  q5=0 m^3/s  q5_nominal_specify=off  q5_nominal_unit=m^3/s  q5_nominal_value=1  q6_specify=off  q6_priority=None  q6=0 m^3/s  q6_nominal_specify=off  q6_nominal_unit=m^3/s  q6_nominal_value=1  qs_specify=off  qs_priority=None  qs=0 m^3/s  qs_nominal_specify=off  qs_nominal_unit=m^3/s  qs_nominal_value=1  qt_specify=off  qt_priority=None  qt=0 m^3/s  qt_nominal_specify=off  qt_nominal_unit=m^3/s  qt_nominal_value=1  p1_specify=off  p1_priority=High  p1=125 bar  p1_nominal_specify=off  p1_nominal_unit=bar  p1_nominal_value=1  p2_specify=off  p2_priority=High  p2=125 bar  p2_nominal_specify=off  p2_nominal_unit=bar  p2_nominal_value=1
  fourway fourland valve1 : fourway_fourland_valve_lib/fourway fourland valve  xv_max=valve_mmorifice_max mm  ps_specify=off  ps_priority=None  ps=0 bar  ps_nominal_specify=off  ps_nominal_unit=bar  ps_nominal_value=1  pt_specify=off  pt_priority=None  pt=0 bar  pt_nominal_specify=off  pt_nominal_unit=bar  pt_nominal_value=1  q1_specify=off  q1_priority=None  q1=0 m^3/s  q1_nominal_specify=off  q1_nominal_unit=m^3/s  q1_nominal_value=1  q2_specify=off  q2_priority=None  q2=0 m^3/s  q2_nominal_specify=off  q2_nominal_unit=m^3/s  q2_nominal_value=1  q3_specify=off  q3_priority=None  q3=0 m^3/s  q3_nominal_specify=off  q3_nominal_unit=m^3/s  q3_nominal_value=1  q4_specify=off  q4_priority=None  q4=0 m^3/s  q4_nominal_specify=off  q4_nominal_unit=m^3/s  q4_nominal_value=1  q5_specify=off  q5_priority=None  q5=0 m^3/s  q5_nominal_specify=off  q5_nominal_unit=m^3/s  q5_nominal_value=1  q6_specify=off  q6_priority=None  q6=0 m^3/s  q6_nominal_specify=off  q6_nominal_unit=m^3/s  q6_nominal_value=1  qs_specify=off  qs_priority=None  qs=0 m^3/s  qs_nominal_specify=off  qs_nominal_unit=m^3/s  qs_nominal_value=1  qt_specify=off  qt_priority=None  qt=0 m^3/s  qt_nominal_specify=off  qt_nominal_unit=m^3/s  qt_nominal_value=1  p1_specify=off  p1_priority=High  p1=125 bar  p1_nominal_specify=off  p1_nominal_unit=bar  p1_nominal_value=1  p2_specify=off  p2_priority=High  p2=125 bar  p2_nominal_specify=off  p2_nominal_unit=bar  p2_nominal_value=1
  p1/p1 : Scope  NumInputPorts=2
      settings: ActiveDisplayYMinimum=-1.5179711239145496E+16  ActiveDisplayYMaximum=1.686657824852189E+15  DataLoggingVariableName=ScopeData3
  p1/p2 : Scope  NumInputPorts=2
      settings: ActiveDisplayYMinimum=25  ActiveDisplayYMaximum=225  DataLoggingVariableName=ScopeData4
  xp/vp : Scope  NumInputPorts=2
      settings: ActiveDisplayYMinimum=-0.0625  ActiveDisplayYMaximum=0.5625
  xp/vp1 : Scope  NumInputPorts=2
      settings: ActiveDisplayYMinimum=-0.07973  ActiveDisplayYMaximum=1.10885  DataLoggingVariableName=ScopeData4
  xp1/xp2 : Scope  NumInputPorts=2
      settings: ActiveDisplayYMinimum=-1  ActiveDisplayYMaximum=1  DataLoggingVariableName=ScopeData5
  xp_re/xp : Scope  NumInputPorts=2
      settings: ActiveDisplayYMinimum=-0.06426  ActiveDisplayYMaximum=0.5627  DataLoggingVariableName=ScopeData7
  ps : PMIOPort  Side=Left
  pt : PMIOPort  Port=2  Side=Left
  load : PMIOPort  Port=3  Side=Right
  wires:
  PS-Simulink Converter3/1 -> p1/p2/1  "p1"
  PS-Simulink Converter7/1 -> controller/2(xp), To Workspace2/1, xp_re/xp/2, xp1/xp2/1, xp/vp/1  "xp"
  PS-Simulink Converter4/1 -> flow/2  "q2"
  PS-Simulink Converter9/1 -> xp/vp/2  "vp"
  PS-Simulink Converter5/1 -> p1/p2/2  "p2"
  PS-Simulink Converter1/1 -> flow/1  "q1"
  PS-Simulink Converter2/1 -> fm/1  "fm"
  PS-Simulink Converter8/1 -> fm1/1  "fm"
  PS-Simulink Converter6/1 -> flow1/1  "q1"
  PS-Simulink Converter12/1 -> p1/p1/2  "p2"
  PS-Simulink Converter14/1 -> xp/vp1/2  "vp"
  PS-Simulink Converter11/1 -> flow1/2  "q2"
  PS-Simulink Converter13/1 -> xp1/xp2/2, xp/vp1/1  "xp"
  PS-Simulink Converter10/1 -> p1/p1/1  "p1"
  ref/1 -> blade_lift_model/1(xp_ref), xp_re/xp/1, To Workspace3/1, controller/1(ref)
  connections:
  bichamber piston A/RConn2 -- PS-Simulink Converter7/LConn1
  bichamber piston A/RConn3 -- PS-Simulink Converter9/LConn1
  bichamber piston A/RConn4 -- PS-Simulink Converter2/LConn1
  bichamber piston A/RConn5 -- PS-Simulink Converter1/LConn1
  bichamber piston A/RConn6 -- PS-Simulink Converter4/LConn1
  bichamber piston A/RConn7 -- PS-Simulink Converter3/LConn1
  bichamber piston A/RConn8 -- PS-Simulink Converter5/LConn1
  bichamber piston A/LConn1 -- fourway fourland valve/RConn1
  bichamber piston A/LConn2 -- fourway fourland valve/RConn2
  ps/RConn1 -- fourway fourland valve1/LConn3 -- fourway fourland valve/LConn3
  pt/RConn1 -- fourway fourland valve1/LConn4 -- fourway fourland valve/LConn4
  controller/RConn1 -- fourway fourland valve1/LConn1 -- fourway fourland valve/LConn1
  PS Constant/RConn1 -- fourway fourland valve/LConn2 -- fourway fourland valve1/LConn2
  bichamber piston B/RConn7 -- PS-Simulink Converter10/LConn1
  bichamber piston B/RConn5 -- PS-Simulink Converter6/LConn1
  bichamber piston B/RConn8 -- PS-Simulink Converter12/LConn1
  bichamber piston B/RConn4 -- PS-Simulink Converter8/LConn1
  bichamber piston B/RConn2 -- PS-Simulink Converter13/LConn1
  bichamber piston B/RConn3 -- PS-Simulink Converter14/LConn1
  bichamber piston B/RConn6 -- PS-Simulink Converter11/LConn1
  fourway fourland valve1/RConn1 -- bichamber piston B/LConn1
  fourway fourland valve1/RConn2 -- bichamber piston B/LConn2
  Connection Label3/LConn1 -- bichamber piston A/RConn1
  Connection Label4/LConn1 -- bichamber piston B/RConn1
  Connection Label1/LConn1 -- blade_lift_model/LConn1
  load/RConn1 -- blade_lift_model/RConn1
  Connection Label2/LConn1 -- blade_lift_model/LConn2
